simulink model "HelicopterNonLinear"  (R2023a)
settings: Solver=VariableStepAuto  StartTime=0.0  StopTime=inf  RelTol=1e-3
values from neighbouring files (symbols this model uses):
  B_p = 0.01    [init.m]
  B_y = 0.08    [init.m]
  g = 9.81    [init.m]
  j_eq_p = 0.0172    [init.m]
  j_eq_y = 0.0210    (= 0.021)    [init.m]
  K_pp = 0.0556    [init.m]
  K_py = 0.005    [init.m]
  K_yp = 0.15    [init.m]
  K_yy = 0.21084    [init.m]
  l_cm = 0.015    [init.m]
  m_heli = 0.479    [init.m]
libraries: simulink_extras x2
settings Model: Creator=Jardar Fagerlund  LastModifiedBy=Jardar Fagerlund

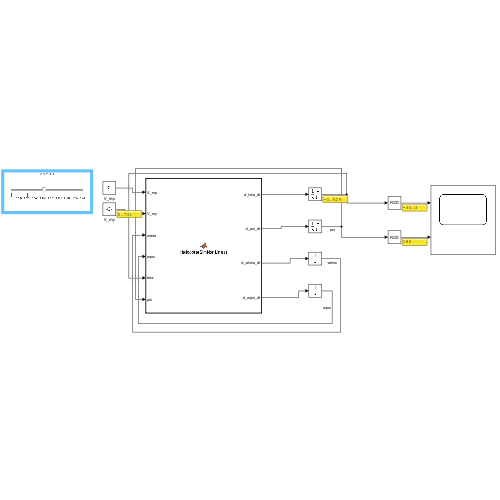
[thumbnail: Simulink's stored preview of the top-level diagram]
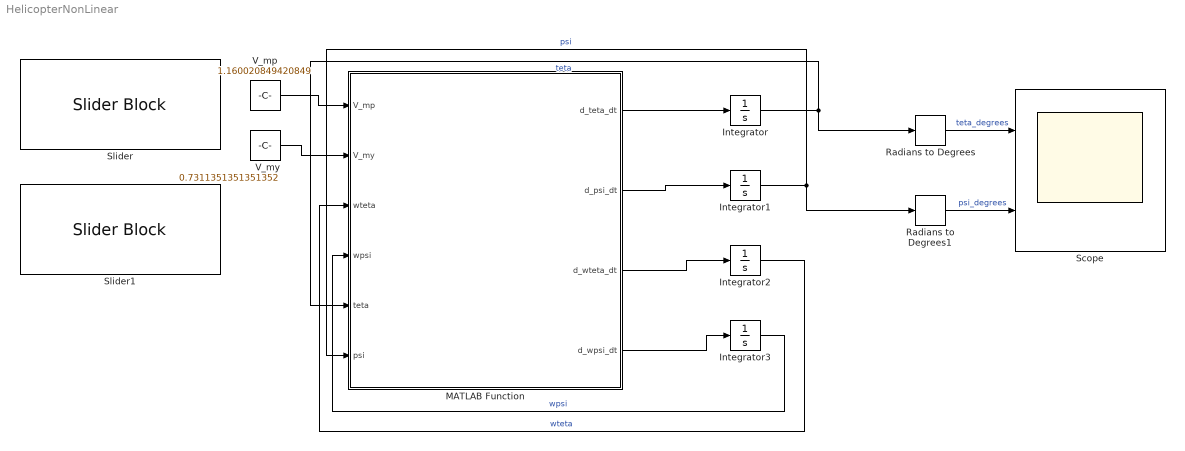
== system HelicopterNonLinear ==
  Integrator : Integrator  InitialCondition=-10*pi/180  LimitOutput=on  UpperSaturationLimit=pi/2  LowerSaturationLimit=-35*pi/180
  Integrator1 : Integrator  InitialCondition=pi/2  LimitOutput=on  UpperSaturationLimit=pi  LowerSaturationLimit=0
  Integrator2 : Integrator
  Integrator3 : Integrator
  MATLAB Function : MATLAB Function  TreatAsAtomicUnit=on
  Radians to Degrees : simulink_extras/Transformations/Radians to Degrees
  Radians to Degrees1 : simulink_extras/Transformations/Radians to Degrees
  Scope : Scope  NumInputPorts=2
  Slider : SliderBlock  ScaleMin=1.1  ScaleMax=1.23
  Slider1 : SliderBlock  ScaleMin=0.4  ScaleMax=1
  V_mp : Constant  Value=1.160020849420849
  V_my : Constant  Value=0.7311351351351352
  wires:
  MATLAB Function/1(d_teta_dt) -> Integrator/1
  MATLAB Function/2(d_psi_dt) -> Integrator1/1
  MATLAB Function/3(d_wteta_dt) -> Integrator2/1
  MATLAB Function/4(d_wpsi_dt) -> Integrator3/1
  Integrator2/1 -> MATLAB Function/3(wteta)  "wteta"
  Integrator3/1 -> MATLAB Function/4(wpsi)  "wpsi"
  Integrator1/1 -> Radians to Degrees1/1, MATLAB Function/6(psi)  "psi"
  Integrator/1 -> Radians to Degrees/1, MATLAB Function/5(teta)  "teta"
  V_mp/1 -> MATLAB Function/1(V_mp)
  V_my/1 -> MATLAB Function/2(V_my)
  Radians to Degrees/1 -> Scope/1  "teta_degrees"
  Radians to Degrees1/1 -> Scope/2  "psi_degrees"

== matlab function HelicopterNonLinear/MATLAB Function ==
  data: V_mp input; d_teta_dt output; V_my input; wteta input; wpsi input; teta input; psi input; d_psi_dt output; d_wteta_dt output; d_wpsi_dt output; K_pp parameter; K_yy parameter; l_cm parameter; m_heli parameter; j_eq_p parameter; j_eq_y parameter; g parameter; K_py parameter; K_yp parameter; B_p parameter; B_y parameter
function [d_teta_dt, d_psi_dt, d_wteta_dt, d_wpsi_dt] = HelicopterSimNonLinear(V_mp, V_my, wteta, wpsi, teta, psi, K_pp,K_yy,l_cm, m_heli, j_eq_p, j_eq_y, g, K_py, K_yp, B_p, B_y)

d_teta_dt = wteta;
d_psi_dt = wpsi;
d_wteta_dt = K_pp*V_mp/(j_eq_p + m_heli*l_cm^2) - K_py*V_my/(j_eq_p + m_heli*l_cm^2) - (B_p*wteta + m_heli*wpsi^2*sin(teta)*l_cm^2*cos(teta)+ m_heli*g*cos(teta)*l_cm)/(j_eq_p + m_heli*l_cm^2);
d_wpsi_dt = K_yp*V_mp/(j_eq_y + m_heli*cos(teta)^2*l_cm^2) - K_yy*V_my/(j_eq_y + m_heli*cos(teta)^2*l_cm^2) + 2*m_heli*wpsi*sin(teta)*l_cm^2*cos(teta)*wteta/(j_eq_y + m_heli*cos(teta)^2*l_cm^2) - B_y*wpsi/(j_eq_y+m_heli*cos(teta)^2*l_cm^2);
